simulink model "Tipo3_v4"  (R2018b)
settings: Solver=FixedStepDiscrete  StartTime=0.0  StopTime=30  MaxStep=50e-6  RelTol=1e-3
PreLoadFcn:
  | Ts=2e-6;
InitFcn:
  | %xInitial = init_power_wind_dfig_det;
  | Ts=2e-6;
undefined symbols (not defined in the file): D1, Delta, DiscIntNeverNeededParam, find_system, level
libraries: powerlib x142, simulink x110, powerlib_meascontrol x63, powerlib_extras x38, simulink_extras x10
(part 3 of 6)

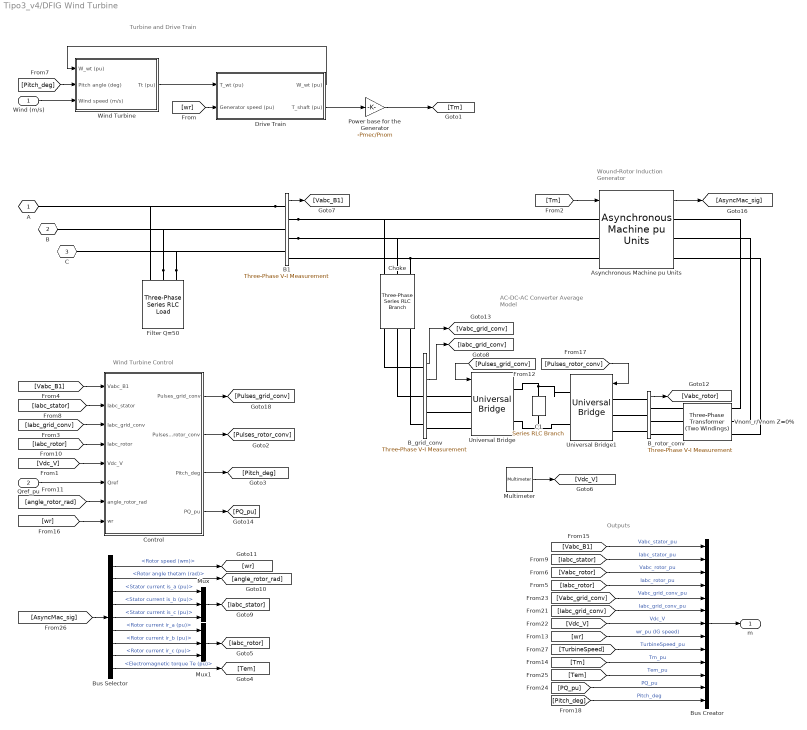
== system Tipo3_v4/DFIG Wind Turbine ==
  note: Turbine and Drive Train
  note: Wind Turbine Control
  note: Wound-Rotor
      | Induction Generator
  note: AC-DC-AC Converter
      | Average Model
  note: Outputs
  "Wind (m/s) " : Inport
  Qref_pu : Inport  Port=2
  Asynchronous Machine pu Units : powerlib/Machines/Asynchronous Machine pu Units  RotorType=Wound  PresetModel=No  MechanicalLoad=Torque Tm  ShowDetailedParameters=on  ReferenceFrame=Rotor  Units=pu  MeasurementBus=off  NominalParameters=[ Pnom Vnom Fnom ]  Stator=[ Rs Lls]  Rotor=[ Rr Llr]  Cage1=[0.01909 0.0397]  Cage2=[0.01909 0.0397]  Lm=Lm  Mechanical=[H F p]  PolePairs=3  InitialConditions=init  SimulateSaturation=off  Saturation="[0.212,0.4201,0.8125,1.0979,1.4799,2.2457,3.2586,4.5763,6.4763 ;   0.5,0.7,0.9,1,1.1,1.2 ,1.3,1.4,1.5]"  LoadFlowParameters=0  TsPowergui=0  TsBlock=-1  IterativeModel=Trapezoidal non iterative  IterativeDiscreteModel=Trapezoidal non iterative  Pmec=0
      settings: SourceProductName=Simscape Electrical  SourceProductBaseCode=PS
  B1 : powerlib/Measurements/Three-Phase V-I Measurement  VoltageMeasurement=phase-to-ground  SetLabelV=off  LabelV=Vabc  Vpu=on  VpuLL=off  CurrentMeasurement=no  SetLabelI=on  LabelI=Iabc_B1  Ipu=on  Pbase=Pnom  Vbase=Vnom  OutputType=Complex  PhasorSimulation=off  PSBequivalent=0
      settings: SourceProductName=Simscape Electrical
  B_grid_conv : powerlib/Measurements/Three-Phase V-I Measurement  VoltageMeasurement=phase-to-ground  SetLabelV=off  LabelV=Vabc_B1  Vpu=on  VpuLL=off  CurrentMeasurement=yes  SetLabelI=off  LabelI=Iabc  Ipu=on  Pbase=Pnom  Vbase=Vnom  OutputType=Complex  PhasorSimulation=off  PSBequivalent=0
      settings: SourceProductName=Simscape Electrical
  B_rotor_conv : powerlib/Measurements/Three-Phase V-I Measurement  VoltageMeasurement=phase-to-phase  SetLabelV=off  LabelV=Vabc_B1  Vpu=on  VpuLL=off  CurrentMeasurement=no  SetLabelI=off  LabelI=Iabc  Ipu=on  Pbase=Pnom  Vbase=Vnom_r  OutputType=Complex  PhasorSimulation=off  PSBequivalent=0
      settings: SourceProductName=Simscape Electrical
  Bus Creator : BusCreator  Inputs=13
  Bus Selector : BusSelector  OutputSignals=Mechanical.Rotor speed (wm),Mechanical.Rotor angle thetam (rad),Stator measurements.Stator current is_a (pu),Stator measurements.Stator current is_b (pu),Stator measurements.Stator current is_c (pu),Rotor measurements.Rotor current ir_a (pu),Rotor measurements.Rotor current ir_b (pu),Rotor measurements.Rotor current ir_c (pu),Mechanical.Electromagnetic torque Te (pu)
  C1 : powerlib/Elements/Series RLC Branch  LConnTagsString=__new0  RConnTagsString=__new0  BranchType=C  Resistance=[]  Inductance=[]  SetiL0=off  InitialCurrent=0  Capacitance=C_DClink  Setx0=on  InitialVoltage=Vdc_nom  Measurements=Branch voltage
      settings: SourceProductName=Simscape Electrical
  "Choke " : powerlib/Elements/Three-Phase Series RLC Branch  LConnTagsString=A|B|C  RConnTagsString=A|B|C  BranchType=RL  Resistance=R_RL*Vnom^2/Pnom  Inductance=L_RL*Vnom^2/Pnom/(2*pi*Fnom)  Capacitance=[]  Measurements=None
      settings: SourceProductName=Simscape Electrical
  Control : Subsystem
  Drive Train : Subsystem  mask(Wind Turbine shaft){H_WT=H_WT, Ksh=Ksh, D_mutual=D_mutual, wbase=2*pi*Fnom/p, w_wt0=w_wt0, torque0=torque0, Ts=Ts}
      mask prompts: H_WT "Wind turbine inertia constant H (s):"; Ksh "Shaft spring constant (pu of nominal mechanical torque/rad):"; D_mutual "Shaft mutual damping (pu of nominal mechanical torque/pu dw):"; wbase "Shaft base speed (rad/s):"; w_wt0 "Turbine initial speed (pu of base speed):"; torque0 "Initial output torque (pu of nominal mechanical torque):"; Ts "Sample time (s):"
      mask help:
      | This block implements a wind turbine drive train model. All shaft parameters are referred to high-speed shaft (generator shaft).
      |
      | The first input is the wind turbine torque in per unit (pu) based on the nominal power of the turbine and the base speed of the generator. The second input is the generator speed in pu based on the base speed of the generator.
      |
      | The outputs are:
      | 1- the transmitted torque of the shaft in pu based on the nominal power of the turbine and the base speed of the generator.
      | 2- the wind turbine speed in pu of the base speed of the generator.
  Filter Q=50 : powerlib/Elements/Three-Phase Series RLC Load  LConnTagsString=A|B|C  Configuration=Y (grounded)  NominalVoltage=Vnom  Vabc=[1e3 1e3 1e3]  Vabcp=[1e3 1e3 1e3]  NominalFrequency=Fnom  UnbalancedPower=off  ActivePower=C_var_filter/Q_filter  InductivePower=0  CapacitivePower=C_var_filter  Pabc=[10e3 9e3 11e3]  QLabc=[100 90 110]  QCabc=[100 90 110]  Pabcp=[10e3 9e3 11e3]  QLabcp=[100 90 110]  QCabcp=[100 90 110]  Measurements=None  LoadType=constant Z
      settings: SourceProductName=Simscape Electrical
  Multimeter : powerlib/Measurements/Multimeter  PhasorSimulation=off  OutputType=Complex  sel=1  L=1  Gain=1  yselected={'Ub: DFIG Wind Turbine/C1'};  PSBOutputType=1  PSBequivalent=0  AxesSetting=[0,0.1,-100,100]  Display=0  SavedBlockNames=-11
      settings: SourceProductName=Simscape Electrical
  Mux : Mux  Inputs=3
  Mux1 : Mux  Inputs=3
  Power base for the Generator : Gain  Gain=-Pmec/Pnom  SaturateOnIntegerOverflow=on  OutDataTypeStr=Inherit: Same as input  ParamDataTypeStr=Inherit: Same as input
  Universal Bridge : powerlib/Power Electronics/Universal Bridge  Arms=3  SnubberResistance=1e3  SnubberCapacitance=inf  Device=IGBT / Diodes  Ron=1e-4/Nb_wt  Lon=0  ForwardVoltages="[  0  0  ]"  ForwardVoltage=0  GTOparameters=[ 10e-6 , 20e-6 ]  IGBTparameters=[ 0 , 0 ]  Measurements=None  Measurements_2=None  converterType=Rectifier
      settings: SourceProductName=Simscape Electrical
  Universal Bridge1 : powerlib/Power Electronics/Universal Bridge  Arms=3  SnubberResistance=1e3  SnubberCapacitance=inf  Device=IGBT / Diodes  Ron=1e-4/Nb_wt  Lon=0  ForwardVoltages="[  0  0  ]"  ForwardVoltage=0  GTOparameters=[ 10e-6 , 20e-6 ]  IGBTparameters=[ 0 , 0 ]  Measurements=None  Measurements_2=None  converterType=Rectifier
      settings: SourceProductName=Simscape Electrical
  Vnom_r/Vnom Z=0% : powerlib/Elements/Three-Phase Transformer (Two Windings)  Winding1Connection=Y  Winding2Connection=Y  CoreType=Three single-phase transformers  SetSaturation=off  Hysteresis=off  DataFile='hysteresis'  SetInitialFlux=off  Measurements=None  UNITS=pu  NominalPower=[ Pnom , Fnom ]  Winding1=[ Vnom_r , 0, 0]  Winding2=[ Vnom , 0, 0]  Rm=500  Lm=inf  L0=0.5  Saturation=[ 0,0 ; 0.0024,1.2 ; 1.0,1.52 ]  InitialFluxes=[ 0.8 , -0.8 , 0.7 ]  MoreParameters=off  BreakLoop=off  DataType=off  TransfoNumber=0
      settings: SourceProductName=Simscape Electrical
  Wind Turbine : Subsystem  mask(Wind Turbine){Prated=Pmec, c1_c8=c1_c8, K1_K2=K1_K2, wind0=wind0, Ts=Ts}
      mask prompts: Prated "Nominal mechanical output power (W):"; c1_c8 "Coefficients [c1 ... c8]"; K1_K2 "Parameters [K1 K2]"; wind0 "Initial wind speed (m/s):"; Ts "Sample time (s):"
      mask help:
      | This block implements a generic wind turbine models.
      |
      | The first input is the turbine speed in per unit of the generator base speed. For a synchronous or asynchronous generator, the base speed is the synchronous speed. For a permanent-magnet generator, the base speed is defined as the speed producing nominal voltage at  no load. The second input is the blade pitch angle in degrees. The third input is the wind speed in m/s.
      |
      | The output is the torque applied to the drive train in per unit based on the nominal power of the turbine and the base speed of the generator.
      mask init:
      | c1 = c1_c8(1);
      | c2 = c1_c8(2);
      | c3 = c1_c8(3);
      | c4 = c1_c8(4);
      | c5 = c1_c8(5);
      | c6 = c1_c8(6);
      | c7 = c1_c8(7);;
      | c8 = c1_c8(8);
      | 
      | K1=K1_K2(1);
      | K2=K1_K2(2);
      settings: OpenFcn=power_openblockproxy();
      mask Display: disp('');
  A : PMIOPort  Tag=PMCPort  Side=Left
  B : PMIOPort  Tag=PMCPort  Port=2  Side=Left
  C : PMIOPort  Tag=PMCPort  Port=3  Side=Left
  m : Outport
  wires:
  [Pulses_rotor_conv] -> Universal Bridge1/1
  [Pulses_grid_conv] -> Universal Bridge/1
  Multimeter/1 -> [Vdc_V]
  [Pitch_deg] -> Bus Creator/13  "Pitch_deg"
  [PQ_pu] -> Bus Creator/12  "PQ_pu"
  Control/4(PQ_pu) -> [PQ_pu]
  [Tem] -> Bus Creator/11  "Tem_pu"
  [Tm] -> Bus Creator/10  "Tm_pu"
  [TurbineSpeed] -> Bus Creator/9  "TurbineSpeed_pu"
  [Vdc_V] -> Bus Creator/7  "Vdc_V"
  [Iabc_grid_conv] -> Bus Creator/6  "Iabc_grid_conv_pu"
  [Vabc_grid_conv] -> Bus Creator/5  "Vabc_grid_conv_pu"
  [Iabc_rotor] -> Bus Creator/4  "Iabc_rotor_pu"
  [Vabc_rotor] -> Bus Creator/3  "Vabc_rotor_pu"
  [Iabc_stator] -> Bus Creator/2  "Iabc_stator_pu"
  [Vabc_B1] -> Bus Creator/1  "Vabc_stator_pu"
  Asynchronous Machine pu Units/1 -> [AsyncMac_sig]
  Control/2(Pulses_rotor_conv) -> [Pulses_rotor_conv]
  [Pitch_deg] -> Wind Turbine/2(Pitch angle (deg))
  Drive Train/1(W_wt (pu)) -> Wind Turbine/1(W_wt (pu))
  "Wind (m/s) "/1 -> Wind Turbine/3(Wind speed (m/s))
  Power base for the Generator/1 -> [Tm]
  Drive Train/2(T_shaft (pu)) -> Power base for the Generator/1
  [wr] -> Drive Train/2(Generator speed (pu))
  Wind Turbine/1(Tt (pu)) -> Drive Train/1(T_wt (pu))
  Qref_pu/1 -> Control/6(Qref)
  Bus Selector/9 -> [Tem]  "<Electromagnetic torque Te (pu)>"
  Bus Selector/1 -> [wr]  "<Rotor speed (wm)>"
  Bus Creator/1 -> m/1
  B_rotor_conv/1 -> [Vabc_rotor]
  B1/1 -> [Vabc_B1]
  [Vabc_B1] -> Control/1(Vabc_B1)
  [Iabc_grid_conv] -> Control/3(Iabc_grid_conv)
  [Iabc_rotor] -> Control/4(Iabc_rotor)
  [angle_rotor_rad] -> Control/7(angle_rotor_rad)
  Mux1/1 -> [Iabc_rotor]
  Mux/1 -> [Iabc_stator]
  [Vdc_V] -> Control/5(Vdc_V)
  Control/3(Pitch_deg) -> [Pitch_deg]
  [Iabc_stator] -> Control/2(Iabc_stator)
  [wr] -> Control/8(wr)
  Bus Selector/8 -> Mux1/3  "<Rotor current ir_c (pu)>"
  Bus Selector/7 -> Mux1/2  "<Rotor current ir_b (pu)>"
  Bus Selector/6 -> Mux1/1  "<Rotor current ir_a (pu)>"
  Bus Selector/5 -> Mux/3  "<Stator current is_c (pu)>"
  Bus Selector/4 -> Mux/2  "<Stator current is_b (pu)>"
  Bus Selector/3 -> Mux/1  "<Stator current is_a (pu)>"
  Bus Selector/2 -> [angle_rotor_rad]  "<Rotor angle thetam (rad)>"
  B_grid_conv/2 -> [Iabc_grid_conv]
  B_grid_conv/1 -> [Vabc_grid_conv]
  Control/1(Pulses_grid_conv) -> [Pulses_grid_conv]
  [AsyncMac_sig] -> Bus Selector/1
  [wr] -> Bus Creator/8  "wr_pu (IG speed)"
  [Tm] -> Asynchronous Machine pu Units/1
  connections:
  Universal Bridge1/LConn3 -- B_rotor_conv/LConn3
  Universal Bridge1/LConn2 -- B_rotor_conv/LConn2
  Universal Bridge1/LConn1 -- B_rotor_conv/LConn1
  C1/LConn1 -- Universal Bridge/RConn1 -- Universal Bridge1/RConn1
  B_grid_conv/RConn2 -- Universal Bridge/LConn2
  B_grid_conv/RConn1 -- Universal Bridge/LConn1
  B_grid_conv/RConn3 -- Universal Bridge/LConn3
  C1/RConn1 -- Universal Bridge/RConn2 -- Universal Bridge1/RConn2
  Filter Q=50/LConn3 -- B1/LConn3 -- C/RConn1
  Filter Q=50/LConn2 -- B1/LConn2 -- B/RConn1
  B1/LConn1 -- Filter Q=50/LConn1 -- A/RConn1
  B_rotor_conv/RConn3 -- Vnom_r/Vnom Z=0%/LConn3
  B_rotor_conv/RConn2 -- Vnom_r/Vnom Z=0%/LConn2
  B_rotor_conv/RConn1 -- Vnom_r/Vnom Z=0%/LConn1
  B1/RConn3 -- "Choke "/LConn3 -- Asynchronous Machine pu Units/LConn3
  B1/RConn1 -- "Choke "/LConn1 -- Asynchronous Machine pu Units/LConn1
  Asynchronous Machine pu Units/RConn3 -- Vnom_r/Vnom Z=0%/RConn3
  Asynchronous Machine pu Units/RConn1 -- Vnom_r/Vnom Z=0%/RConn1
  Asynchronous Machine pu Units/RConn2 -- Vnom_r/Vnom Z=0%/RConn2
  "Choke "/RConn3 -- B_grid_conv/LConn3
  "Choke "/RConn2 -- B_grid_conv/LConn2
  "Choke "/RConn1 -- B_grid_conv/LConn1
  B1/RConn2 -- "Choke "/LConn2 -- Asynchronous Machine pu Units/LConn2

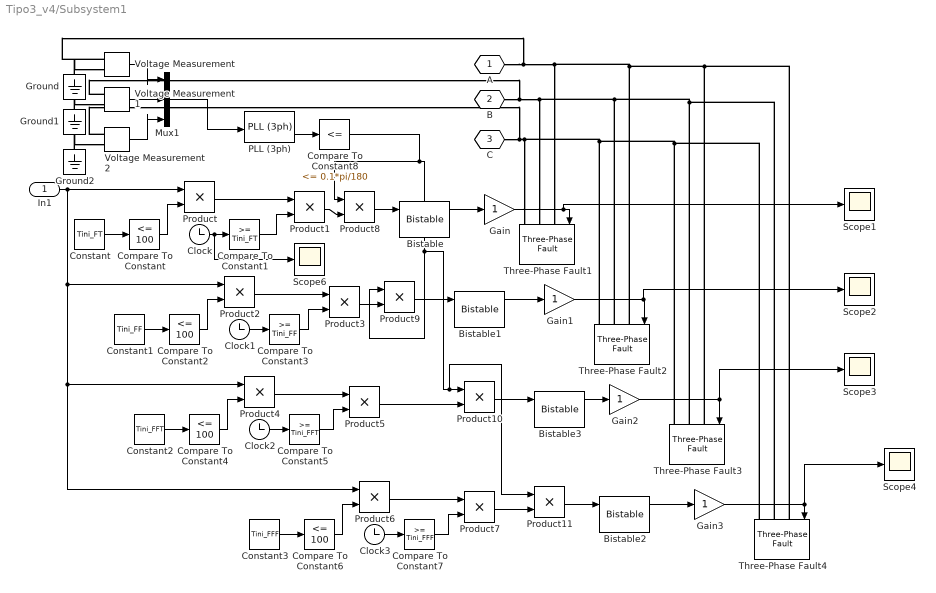
== system Tipo3_v4/Subsystem1 ==
  In1 : Inport
  Bistable{,1..3} (4 alike) : powerlib_meascontrol/Logic/Bistable  Qpriority=Set  ic=0  Ts=Ts
      settings: SourceProductName=Simscape Power Systems  SourceProductBaseCode=PS
  Clock{,1..3} (4 alike) : Clock
  Compare To Constant{,2,4,6} (4 alike) : simulink/Logic and Bit Operations/Compare To Constant  relop=<=  const=100  OutDataTypeStr=uint8
  Compare To Constant1 : simulink/Logic and Bit Operations/Compare To Constant  relop=>=  const=Tini_FT  OutDataTypeStr=uint8
  Compare To Constant3 : simulink/Logic and Bit Operations/Compare To Constant  relop=>=  const=Tini_FF  OutDataTypeStr=uint8
  Compare To Constant5 : simulink/Logic and Bit Operations/Compare To Constant  relop=>=  const=Tini_FFT  OutDataTypeStr=uint8
  Compare To Constant7 : simulink/Logic and Bit Operations/Compare To Constant  relop=>=  const=Tini_FFF  OutDataTypeStr=uint8
  Compare To Constant8 : simulink/Logic and Bit Operations/Compare To Constant  relop=<=  const=0.1*pi/180  OutDataTypeStr=uint8
  Constant : Constant  Value=Tini_FT
  Constant1 : Constant  Value=Tini_FF
  Constant2 : Constant  Value=Tini_FFT
  Constant3 : Constant  Value=Tini_FFF
  Gain{,1..3} (4 alike) : Gain  OutDataTypeStr=double
  Ground : powerlib/Elements/Ground  LConnTagsString=a
  Ground1 : powerlib/Elements/Ground  LConnTagsString=a
  Ground2 : powerlib/Elements/Ground  LConnTagsString=a
  Mux1 : Mux  Inputs=3
  PLL (3ph) : powerlib_meascontrol/PLL/PLL (3ph)  Fmin=60  Par_Init=[0, 60]  ParK=[180, 3200, 1]  TcD=1e-4  MaxRateChangeFreq=12  FilterCutOffFreq=25  Ts=Ts  AGC=on
  Product{,2..7} (7 alike) : Product
  Product{1,8..11} (5 alike) : Product  RndMeth=Ceiling
  Scope{1..4,6} (5 alike) : Scope
  Three-Phase Fault1 : powerlib/Elements/Three-Phase Fault  InitialStates=0  FaultA=on  FaultB=off  FaultC=off  GroundFault=on  SwitchTimes=[900 1000]  External=on  SwitchStatus=NaN  FaultResistance=R_falta  GroundResistance=R_falta  SnubberResistance=1e6  SnubberCapacitance=inf  Measurements=None
  Three-Phase Fault2 : powerlib/Elements/Three-Phase Fault  InitialStates=0  FaultA=on  FaultB=on  FaultC=off  GroundFault=off  SwitchTimes=[900 1000]  External=on  SwitchStatus=NaN  FaultResistance=R_falta  GroundResistance=1e-12  SnubberResistance=1e6  SnubberCapacitance=inf  Measurements=None
  Three-Phase Fault3 : powerlib/Elements/Three-Phase Fault  InitialStates=0  FaultA=on  FaultB=on  FaultC=off  GroundFault=on  SwitchTimes=[900 1000]  External=on  SwitchStatus=NaN  FaultResistance=R_falta  GroundResistance=R_falta  SnubberResistance=1e6  SnubberCapacitance=inf  Measurements=None
  Three-Phase Fault4 : powerlib/Elements/Three-Phase Fault  InitialStates=0  FaultA=on  FaultB=on  FaultC=on  GroundFault=on  SwitchTimes=[900 1000]  External=on  SwitchStatus=NaN  FaultResistance=R_falta  GroundResistance=R_falta  SnubberResistance=1e6  SnubberCapacitance=inf  Measurements=None
  Voltage Measurement : powerlib/Measurements/Voltage Measurement  PhasorSimulation=off  OutputType=Complex  PSBequivalent=0
  Voltage Measurement1 : powerlib/Measurements/Voltage Measurement  PhasorSimulation=off  OutputType=Complex  PSBequivalent=0
  Voltage Measurement2 : powerlib/Measurements/Voltage Measurement  PhasorSimulation=off  OutputType=Complex  PSBequivalent=0
  A : PMIOPort  Tag=PMCPort  Side=Right
  B : PMIOPort  Tag=PMCPort  Port=2  Side=Right
  C : PMIOPort  Tag=PMCPort  Port=3  Side=Right
  wires:
  Clock/1 -> Scope6/1, Compare To Constant1/1
  Product2/1 -> Product3/1
  Constant1/1 -> Compare To Constant2/1
  Product/1 -> Product1/1
  Compare To Constant2/1 -> Product2/2
  Constant2/1 -> Compare To Constant4/1
  Clock2/1 -> Compare To Constant5/1
  Compare To Constant4/1 -> Product4/2
  Clock1/1 -> Compare To Constant3/1
  Compare To Constant5/1 -> Product5/2
  In1/1 -> Product/1, Product2/1, Product4/1, Product6/1
  Clock3/1 -> Compare To Constant7/1
  Constant3/1 -> Compare To Constant6/1
  Compare To Constant6/1 -> Product6/2
  Product6/1 -> Product7/1
  Compare To Constant7/1 -> Product7/2
  Compare To Constant3/1 -> Product3/2
  Constant/1 -> Compare To Constant/1
  Compare To Constant/1 -> Product/2
  Compare To Constant1/1 -> Product1/2
  Product4/1 -> Product5/1
  Product1/1 -> Product8/2
  Product8/1 -> Bistable/1
  Product3/1 -> Product9/2
  Product5/1 -> Product10/2
  Product7/1 -> Product11/2
  Compare To Constant8/1 -> Product11/1, Product10/1, Product9/1, Product8/1
  PLL (3ph)/2 -> Compare To Constant8/1
  Voltage Measurement1/1 -> Mux1/2
  Voltage Measurement/1 -> Mux1/1
  Voltage Measurement2/1 -> Mux1/3
  Mux1/1 -> PLL (3ph)/1
  Gain/1 -> Scope1/1, Three-Phase Fault1/1
  Gain1/1 -> Scope2/1, Three-Phase Fault2/1
  Gain2/1 -> Three-Phase Fault3/1, Scope3/1
  Gain3/1 -> Scope4/1, Three-Phase Fault4/1
  Bistable/1 -> Gain/1
  Product9/1 -> Bistable1/1
  Bistable1/1 -> Gain1/1
  Bistable3/1 -> Gain2/1
  Product10/1 -> Bistable3/1
  Product11/1 -> Bistable2/1
  Bistable2/1 -> Gain3/1
  connections:
  Three-Phase Fault1/LConn2 -- Voltage Measurement1/LConn1 -- B/RConn1 -- Three-Phase Fault2/LConn2 -- Three-Phase Fault3/LConn2 -- Three-Phase Fault4/LConn2
  Three-Phase Fault1/LConn3 -- Voltage Measurement2/LConn1 -- C/RConn1 -- Three-Phase Fault4/LConn3 -- Three-Phase Fault3/LConn3 -- Three-Phase Fault2/LConn3
  A/RConn1 -- Voltage Measurement/LConn1 -- Three-Phase Fault2/LConn1 -- Three-Phase Fault3/LConn1 -- Three-Phase Fault4/LConn1 -- Three-Phase Fault1/LConn1
  Ground/LConn1 -- Voltage Measurement/LConn2
  Ground1/LConn1 -- Voltage Measurement1/LConn2
  Ground2/LConn1 -- Voltage Measurement2/LConn2

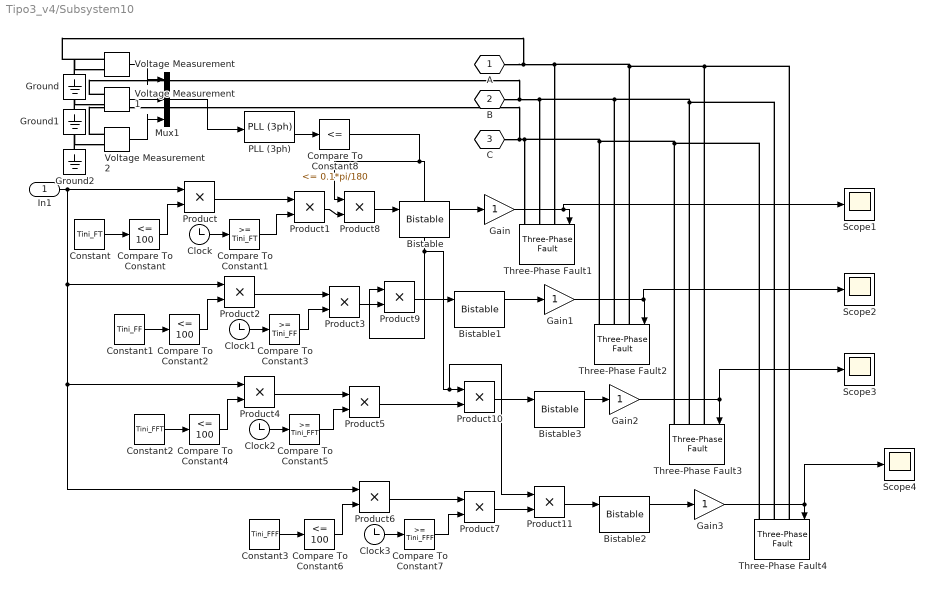
== system Tipo3_v4/Subsystem10 ==
  In1 : Inport
  Bistable{,1..3} (4 alike) : powerlib_meascontrol/Logic/Bistable  Qpriority=Set  ic=0  Ts=Ts
      settings: SourceProductName=Simscape Power Systems  SourceProductBaseCode=PS
  Clock{,1..3} (4 alike) : Clock
  Compare To Constant{,2,4,6} (4 alike) : simulink/Logic and Bit Operations/Compare To Constant  relop=<=  const=100  OutDataTypeStr=uint8
  Compare To Constant1 : simulink/Logic and Bit Operations/Compare To Constant  relop=>=  const=Tini_FT  OutDataTypeStr=uint8
  Compare To Constant3 : simulink/Logic and Bit Operations/Compare To Constant  relop=>=  const=Tini_FF  OutDataTypeStr=uint8
  Compare To Constant5 : simulink/Logic and Bit Operations/Compare To Constant  relop=>=  const=Tini_FFT  OutDataTypeStr=uint8
  Compare To Constant7 : simulink/Logic and Bit Operations/Compare To Constant  relop=>=  const=Tini_FFF  OutDataTypeStr=uint8
  Compare To Constant8 : simulink/Logic and Bit Operations/Compare To Constant  relop=<=  const=0.1*pi/180  OutDataTypeStr=uint8
  Constant : Constant  Value=Tini_FT
  Constant1 : Constant  Value=Tini_FF
  Constant2 : Constant  Value=Tini_FFT
  Constant3 : Constant  Value=Tini_FFF
  Gain{,1..3} (4 alike) : Gain  OutDataTypeStr=double
  Ground : powerlib/Elements/Ground  LConnTagsString=a
  Ground1 : powerlib/Elements/Ground  LConnTagsString=a
  Ground2 : powerlib/Elements/Ground  LConnTagsString=a
  Mux1 : Mux  Inputs=3
  PLL (3ph) : powerlib_meascontrol/PLL/PLL (3ph)  Fmin=60  Par_Init=[0, 60]  ParK=[180, 3200, 1]  TcD=1e-4  MaxRateChangeFreq=12  FilterCutOffFreq=25  Ts=Ts  AGC=on
  Product{,2..7} (7 alike) : Product
  Product{1,8..11} (5 alike) : Product  RndMeth=Ceiling
  Scope{1..4} (4 alike) : Scope
  Three-Phase Fault1 : powerlib/Elements/Three-Phase Fault  InitialStates=0  FaultA=on  FaultB=off  FaultC=off  GroundFault=on  SwitchTimes=[900 1000]  External=on  SwitchStatus=NaN  FaultResistance=R_falta  GroundResistance=R_falta  SnubberResistance=1e6  SnubberCapacitance=inf  Measurements=None
  Three-Phase Fault2 : powerlib/Elements/Three-Phase Fault  InitialStates=0  FaultA=on  FaultB=on  FaultC=off  GroundFault=off  SwitchTimes=[900 1000]  External=on  SwitchStatus=NaN  FaultResistance=R_falta  GroundResistance=1e-12  SnubberResistance=1e6  SnubberCapacitance=inf  Measurements=None
  Three-Phase Fault3 : powerlib/Elements/Three-Phase Fault  InitialStates=0  FaultA=on  FaultB=on  FaultC=off  GroundFault=on  SwitchTimes=[900 1000]  External=on  SwitchStatus=NaN  FaultResistance=R_falta  GroundResistance=R_falta  SnubberResistance=1e6  SnubberCapacitance=inf  Measurements=None
  Three-Phase Fault4 : powerlib/Elements/Three-Phase Fault  InitialStates=0  FaultA=on  FaultB=on  FaultC=on  GroundFault=on  SwitchTimes=[900 1000]  External=on  SwitchStatus=NaN  FaultResistance=R_falta  GroundResistance=R_falta  SnubberResistance=1e6  SnubberCapacitance=inf  Measurements=None
  Voltage Measurement : powerlib/Measurements/Voltage Measurement  PhasorSimulation=off  OutputType=Complex  PSBequivalent=0
  Voltage Measurement1 : powerlib/Measurements/Voltage Measurement  PhasorSimulation=off  OutputType=Complex  PSBequivalent=0
  Voltage Measurement2 : powerlib/Measurements/Voltage Measurement  PhasorSimulation=off  OutputType=Complex  PSBequivalent=0
  A : PMIOPort  Tag=PMCPort  Side=Right
  B : PMIOPort  Tag=PMCPort  Port=2  Side=Right
  C : PMIOPort  Tag=PMCPort  Port=3  Side=Right
  wires:
  Clock/1 -> Compare To Constant1/1
  Product2/1 -> Product3/1
  Constant1/1 -> Compare To Constant2/1
  Product/1 -> Product1/1
  Compare To Constant2/1 -> Product2/2
  Constant2/1 -> Compare To Constant4/1
  Clock2/1 -> Compare To Constant5/1
  Compare To Constant4/1 -> Product4/2
  Clock1/1 -> Compare To Constant3/1
  Compare To Constant5/1 -> Product5/2
  In1/1 -> Product/1, Product2/1, Product4/1, Product6/1
  Clock3/1 -> Compare To Constant7/1
  Constant3/1 -> Compare To Constant6/1
  Compare To Constant6/1 -> Product6/2
  Product6/1 -> Product7/1
  Compare To Constant7/1 -> Product7/2
  Compare To Constant3/1 -> Product3/2
  Constant/1 -> Compare To Constant/1
  Compare To Constant/1 -> Product/2
  Compare To Constant1/1 -> Product1/2
  Product4/1 -> Product5/1
  Product1/1 -> Product8/2
  Product8/1 -> Bistable/1
  Product3/1 -> Product9/2
  Product5/1 -> Product10/2
  Product7/1 -> Product11/2
  Compare To Constant8/1 -> Product11/1, Product10/1, Product9/1, Product8/1
  PLL (3ph)/2 -> Compare To Constant8/1
  Voltage Measurement1/1 -> Mux1/2
  Voltage Measurement/1 -> Mux1/1
  Voltage Measurement2/1 -> Mux1/3
  Mux1/1 -> PLL (3ph)/1
  Gain/1 -> Scope1/1, Three-Phase Fault1/1
  Gain1/1 -> Scope2/1, Three-Phase Fault2/1
  Gain2/1 -> Three-Phase Fault3/1, Scope3/1
  Gain3/1 -> Scope4/1, Three-Phase Fault4/1
  Bistable/1 -> Gain/1
  Product9/1 -> Bistable1/1
  Bistable1/1 -> Gain1/1
  Bistable3/1 -> Gain2/1
  Product10/1 -> Bistable3/1
  Product11/1 -> Bistable2/1
  Bistable2/1 -> Gain3/1
  connections:
  Voltage Measurement1/LConn1 -- B/RConn1 -- Three-Phase Fault1/LConn2 -- Three-Phase Fault2/LConn2 -- Three-Phase Fault3/LConn2 -- Three-Phase Fault4/LConn2
  Voltage Measurement2/LConn1 -- C/RConn1 -- Three-Phase Fault4/LConn3 -- Three-Phase Fault3/LConn3 -- Three-Phase Fault2/LConn3 -- Three-Phase Fault1/LConn3
  A/RConn1 -- Voltage Measurement/LConn1 -- Three-Phase Fault1/LConn1 -- Three-Phase Fault2/LConn1 -- Three-Phase Fault3/LConn1 -- Three-Phase Fault4/LConn1
  Ground/LConn1 -- Voltage Measurement/LConn2
  Ground1/LConn1 -- Voltage Measurement1/LConn2
  Ground2/LConn1 -- Voltage Measurement2/LConn2

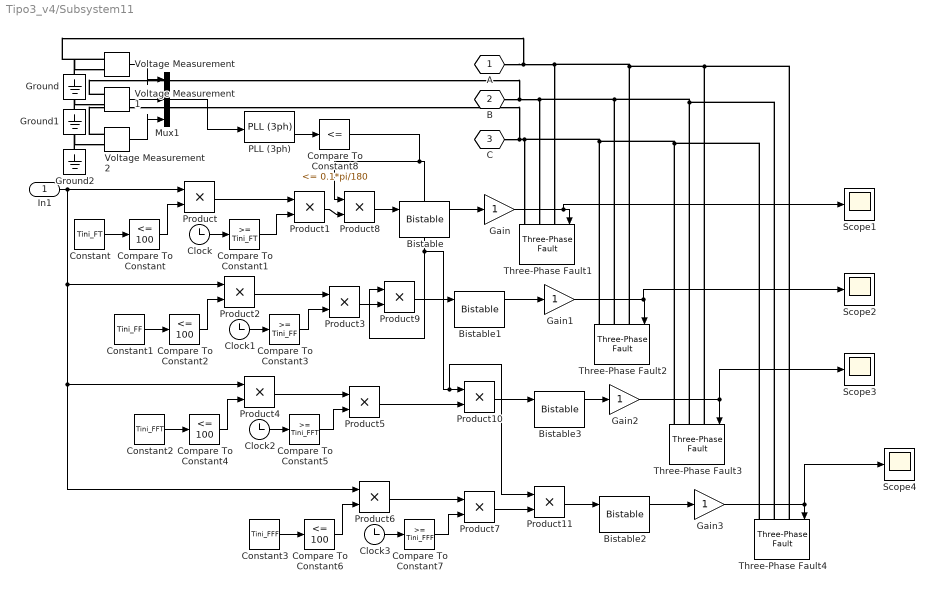
== system Tipo3_v4/Subsystem11 ==
  In1 : Inport
  Bistable{,1..3} (4 alike) : powerlib_meascontrol/Logic/Bistable  Qpriority=Set  ic=0  Ts=Ts
      settings: SourceProductName=Simscape Power Systems  SourceProductBaseCode=PS
  Clock{,1..3} (4 alike) : Clock
  Compare To Constant{,2,4,6} (4 alike) : simulink/Logic and Bit Operations/Compare To Constant  relop=<=  const=100  OutDataTypeStr=uint8
  Compare To Constant1 : simulink/Logic and Bit Operations/Compare To Constant  relop=>=  const=Tini_FT  OutDataTypeStr=uint8
  Compare To Constant3 : simulink/Logic and Bit Operations/Compare To Constant  relop=>=  const=Tini_FF  OutDataTypeStr=uint8
  Compare To Constant5 : simulink/Logic and Bit Operations/Compare To Constant  relop=>=  const=Tini_FFT  OutDataTypeStr=uint8
  Compare To Constant7 : simulink/Logic and Bit Operations/Compare To Constant  relop=>=  const=Tini_FFF  OutDataTypeStr=uint8
  Compare To Constant8 : simulink/Logic and Bit Operations/Compare To Constant  relop=<=  const=0.1*pi/180  OutDataTypeStr=uint8
  Constant : Constant  Value=Tini_FT
  Constant1 : Constant  Value=Tini_FF
  Constant2 : Constant  Value=Tini_FFT
  Constant3 : Constant  Value=Tini_FFF
  Gain{,1..3} (4 alike) : Gain  OutDataTypeStr=double
  Ground : powerlib/Elements/Ground  LConnTagsString=a
  Ground1 : powerlib/Elements/Ground  LConnTagsString=a
  Ground2 : powerlib/Elements/Ground  LConnTagsString=a
  Mux1 : Mux  Inputs=3
  PLL (3ph) : powerlib_meascontrol/PLL/PLL (3ph)  Fmin=60  Par_Init=[0, 60]  ParK=[180, 3200, 1]  TcD=1e-4  MaxRateChangeFreq=12  FilterCutOffFreq=25  Ts=Ts  AGC=on
  Product{,2..7} (7 alike) : Product
  Product{1,8..11} (5 alike) : Product  RndMeth=Ceiling
  Scope{1..4} (4 alike) : Scope
  Three-Phase Fault1 : powerlib/Elements/Three-Phase Fault  InitialStates=0  FaultA=on  FaultB=off  FaultC=off  GroundFault=on  SwitchTimes=[900 1000]  External=on  SwitchStatus=NaN  FaultResistance=R_falta  GroundResistance=R_falta  SnubberResistance=1e6  SnubberCapacitance=inf  Measurements=None
  Three-Phase Fault2 : powerlib/Elements/Three-Phase Fault  InitialStates=0  FaultA=on  FaultB=on  FaultC=off  GroundFault=off  SwitchTimes=[900 1000]  External=on  SwitchStatus=NaN  FaultResistance=R_falta  GroundResistance=1e-12  SnubberResistance=1e6  SnubberCapacitance=inf  Measurements=None
  Three-Phase Fault3 : powerlib/Elements/Three-Phase Fault  InitialStates=0  FaultA=on  FaultB=on  FaultC=off  GroundFault=on  SwitchTimes=[900 1000]  External=on  SwitchStatus=NaN  FaultResistance=R_falta  GroundResistance=R_falta  SnubberResistance=1e6  SnubberCapacitance=inf  Measurements=None
  Three-Phase Fault4 : powerlib/Elements/Three-Phase Fault  InitialStates=0  FaultA=on  FaultB=on  FaultC=on  GroundFault=on  SwitchTimes=[900 1000]  External=on  SwitchStatus=NaN  FaultResistance=R_falta  GroundResistance=R_falta  SnubberResistance=1e6  SnubberCapacitance=inf  Measurements=None
  Voltage Measurement : powerlib/Measurements/Voltage Measurement  PhasorSimulation=off  OutputType=Complex  PSBequivalent=0
  Voltage Measurement1 : powerlib/Measurements/Voltage Measurement  PhasorSimulation=off  OutputType=Complex  PSBequivalent=0
  Voltage Measurement2 : powerlib/Measurements/Voltage Measurement  PhasorSimulation=off  OutputType=Complex  PSBequivalent=0
  A : PMIOPort  Tag=PMCPort  Side=Right
  B : PMIOPort  Tag=PMCPort  Port=2  Side=Right
  C : PMIOPort  Tag=PMCPort  Port=3  Side=Right
  wires:
  Clock/1 -> Compare To Constant1/1
  Product2/1 -> Product3/1
  Constant1/1 -> Compare To Constant2/1
  Product/1 -> Product1/1
  Compare To Constant2/1 -> Product2/2
  Constant2/1 -> Compare To Constant4/1
  Clock2/1 -> Compare To Constant5/1
  Compare To Constant4/1 -> Product4/2
  Clock1/1 -> Compare To Constant3/1
  Compare To Constant5/1 -> Product5/2
  In1/1 -> Product/1, Product2/1, Product4/1, Product6/1
  Clock3/1 -> Compare To Constant7/1
  Constant3/1 -> Compare To Constant6/1
  Compare To Constant6/1 -> Product6/2
  Product6/1 -> Product7/1
  Compare To Constant7/1 -> Product7/2
  Compare To Constant3/1 -> Product3/2
  Constant/1 -> Compare To Constant/1
  Compare To Constant/1 -> Product/2
  Compare To Constant1/1 -> Product1/2
  Product4/1 -> Product5/1
  Product1/1 -> Product8/2
  Product8/1 -> Bistable/1
  Product3/1 -> Product9/2
  Product5/1 -> Product10/2
  Product7/1 -> Product11/2
  Compare To Constant8/1 -> Product11/1, Product10/1, Product9/1, Product8/1
  PLL (3ph)/2 -> Compare To Constant8/1
  Voltage Measurement1/1 -> Mux1/2
  Voltage Measurement/1 -> Mux1/1
  Voltage Measurement2/1 -> Mux1/3
  Mux1/1 -> PLL (3ph)/1
  Gain/1 -> Scope1/1, Three-Phase Fault1/1
  Gain1/1 -> Scope2/1, Three-Phase Fault2/1
  Gain2/1 -> Three-Phase Fault3/1, Scope3/1
  Gain3/1 -> Scope4/1, Three-Phase Fault4/1
  Bistable/1 -> Gain/1
  Product9/1 -> Bistable1/1
  Bistable1/1 -> Gain1/1
  Bistable3/1 -> Gain2/1
  Product10/1 -> Bistable3/1
  Product11/1 -> Bistable2/1
  Bistable2/1 -> Gain3/1
  connections:
  Voltage Measurement1/LConn1 -- B/RConn1 -- Three-Phase Fault1/LConn2 -- Three-Phase Fault2/LConn2 -- Three-Phase Fault3/LConn2 -- Three-Phase Fault4/LConn2
  Voltage Measurement2/LConn1 -- C/RConn1 -- Three-Phase Fault4/LConn3 -- Three-Phase Fault3/LConn3 -- Three-Phase Fault2/LConn3 -- Three-Phase Fault1/LConn3
  A/RConn1 -- Voltage Measurement/LConn1 -- Three-Phase Fault1/LConn1 -- Three-Phase Fault2/LConn1 -- Three-Phase Fault3/LConn1 -- Three-Phase Fault4/LConn1
  Ground/LConn1 -- Voltage Measurement/LConn2
  Ground1/LConn1 -- Voltage Measurement1/LConn2
  Ground2/LConn1 -- Voltage Measurement2/LConn2

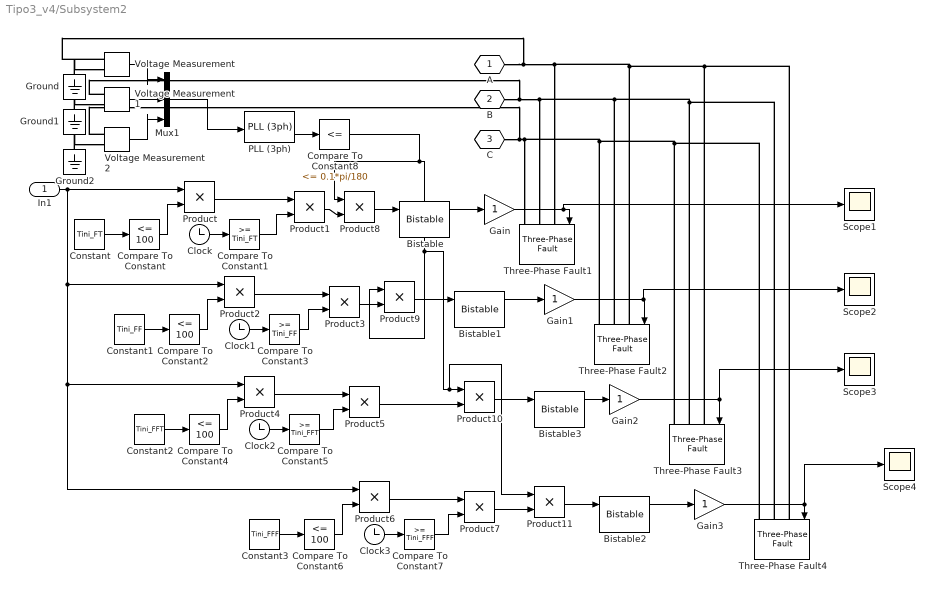
== system Tipo3_v4/Subsystem2 ==
  In1 : Inport
  Bistable{,1..3} (4 alike) : powerlib_meascontrol/Logic/Bistable  Qpriority=Set  ic=0  Ts=Ts
      settings: SourceProductName=Simscape Power Systems  SourceProductBaseCode=PS
  Clock{,1..3} (4 alike) : Clock
  Compare To Constant{,2,4,6} (4 alike) : simulink/Logic and Bit Operations/Compare To Constant  relop=<=  const=100  OutDataTypeStr=uint8
  Compare To Constant1 : simulink/Logic and Bit Operations/Compare To Constant  relop=>=  const=Tini_FT  OutDataTypeStr=uint8
  Compare To Constant3 : simulink/Logic and Bit Operations/Compare To Constant  relop=>=  const=Tini_FF  OutDataTypeStr=uint8
  Compare To Constant5 : simulink/Logic and Bit Operations/Compare To Constant  relop=>=  const=Tini_FFT  OutDataTypeStr=uint8
  Compare To Constant7 : simulink/Logic and Bit Operations/Compare To Constant  relop=>=  const=Tini_FFF  OutDataTypeStr=uint8
  Compare To Constant8 : simulink/Logic and Bit Operations/Compare To Constant  relop=<=  const=0.1*pi/180  OutDataTypeStr=uint8
  Constant : Constant  Value=Tini_FT
  Constant1 : Constant  Value=Tini_FF
  Constant2 : Constant  Value=Tini_FFT
  Constant3 : Constant  Value=Tini_FFF
  Gain{,1..3} (4 alike) : Gain  OutDataTypeStr=double
  Ground : powerlib/Elements/Ground  LConnTagsString=a
  Ground1 : powerlib/Elements/Ground  LConnTagsString=a
  Ground2 : powerlib/Elements/Ground  LConnTagsString=a
  Mux1 : Mux  Inputs=3
  PLL (3ph) : powerlib_meascontrol/PLL/PLL (3ph)  Fmin=60  Par_Init=[0, 60]  ParK=[180, 3200, 1]  TcD=1e-4  MaxRateChangeFreq=12  FilterCutOffFreq=25  Ts=Ts  AGC=on
  Product{,2..7} (7 alike) : Product
  Product{1,8..11} (5 alike) : Product  RndMeth=Ceiling
  Scope{1..4} (4 alike) : Scope
  Three-Phase Fault1 : powerlib/Elements/Three-Phase Fault  InitialStates=0  FaultA=on  FaultB=off  FaultC=off  GroundFault=on  SwitchTimes=[900 1000]  External=on  SwitchStatus=NaN  FaultResistance=R_falta  GroundResistance=R_falta  SnubberResistance=1e6  SnubberCapacitance=inf  Measurements=None
  Three-Phase Fault2 : powerlib/Elements/Three-Phase Fault  InitialStates=0  FaultA=on  FaultB=on  FaultC=off  GroundFault=off  SwitchTimes=[900 1000]  External=on  SwitchStatus=NaN  FaultResistance=R_falta  GroundResistance=1e-12  SnubberResistance=1e6  SnubberCapacitance=inf  Measurements=None
  Three-Phase Fault3 : powerlib/Elements/Three-Phase Fault  InitialStates=0  FaultA=on  FaultB=on  FaultC=off  GroundFault=on  SwitchTimes=[900 1000]  External=on  SwitchStatus=NaN  FaultResistance=R_falta  GroundResistance=R_falta  SnubberResistance=1e6  SnubberCapacitance=inf  Measurements=None
  Three-Phase Fault4 : powerlib/Elements/Three-Phase Fault  InitialStates=0  FaultA=on  FaultB=on  FaultC=on  GroundFault=on  SwitchTimes=[900 1000]  External=on  SwitchStatus=NaN  FaultResistance=R_falta  GroundResistance=R_falta  SnubberResistance=1e6  SnubberCapacitance=inf  Measurements=None
  Voltage Measurement : powerlib/Measurements/Voltage Measurement  PhasorSimulation=off  OutputType=Complex  PSBequivalent=0
  Voltage Measurement1 : powerlib/Measurements/Voltage Measurement  PhasorSimulation=off  OutputType=Complex  PSBequivalent=0
  Voltage Measurement2 : powerlib/Measurements/Voltage Measurement  PhasorSimulation=off  OutputType=Complex  PSBequivalent=0
  A : PMIOPort  Tag=PMCPort  Side=Right
  B : PMIOPort  Tag=PMCPort  Port=2  Side=Right
  C : PMIOPort  Tag=PMCPort  Port=3  Side=Right
  wires:
  Clock/1 -> Compare To Constant1/1
  Product2/1 -> Product3/1
  Constant1/1 -> Compare To Constant2/1
  Product/1 -> Product1/1
  Compare To Constant2/1 -> Product2/2
  Constant2/1 -> Compare To Constant4/1
  Clock2/1 -> Compare To Constant5/1
  Compare To Constant4/1 -> Product4/2
  Clock1/1 -> Compare To Constant3/1
  Compare To Constant5/1 -> Product5/2
  In1/1 -> Product/1, Product2/1, Product4/1, Product6/1
  Clock3/1 -> Compare To Constant7/1
  Constant3/1 -> Compare To Constant6/1
  Compare To Constant6/1 -> Product6/2
  Product6/1 -> Product7/1
  Compare To Constant7/1 -> Product7/2
  Compare To Constant3/1 -> Product3/2
  Constant/1 -> Compare To Constant/1
  Compare To Constant/1 -> Product/2
  Compare To Constant1/1 -> Product1/2
  Product4/1 -> Product5/1
  Product1/1 -> Product8/2
  Product8/1 -> Bistable/1
  Product3/1 -> Product9/2
  Product5/1 -> Product10/2
  Product7/1 -> Product11/2
  Compare To Constant8/1 -> Product11/1, Product10/1, Product9/1, Product8/1
  PLL (3ph)/2 -> Compare To Constant8/1
  Voltage Measurement1/1 -> Mux1/2
  Voltage Measurement/1 -> Mux1/1
  Voltage Measurement2/1 -> Mux1/3
  Mux1/1 -> PLL (3ph)/1
  Gain/1 -> Scope1/1, Three-Phase Fault1/1
  Gain1/1 -> Scope2/1, Three-Phase Fault2/1
  Gain2/1 -> Three-Phase Fault3/1, Scope3/1
  Gain3/1 -> Scope4/1, Three-Phase Fault4/1
  Bistable/1 -> Gain/1
  Product9/1 -> Bistable1/1
  Bistable1/1 -> Gain1/1
  Bistable3/1 -> Gain2/1
  Product10/1 -> Bistable3/1
  Product11/1 -> Bistable2/1
  Bistable2/1 -> Gain3/1
  connections:
  Voltage Measurement1/LConn1 -- B/RConn1 -- Three-Phase Fault1/LConn2 -- Three-Phase Fault2/LConn2 -- Three-Phase Fault3/LConn2 -- Three-Phase Fault4/LConn2
  Voltage Measurement2/LConn1 -- C/RConn1 -- Three-Phase Fault4/LConn3 -- Three-Phase Fault3/LConn3 -- Three-Phase Fault2/LConn3 -- Three-Phase Fault1/LConn3
  A/RConn1 -- Voltage Measurement/LConn1 -- Three-Phase Fault1/LConn1 -- Three-Phase Fault2/LConn1 -- Three-Phase Fault3/LConn1 -- Three-Phase Fault4/LConn1
  Ground/LConn1 -- Voltage Measurement/LConn2
  Ground1/LConn1 -- Voltage Measurement1/LConn2
  Ground2/LConn1 -- Voltage Measurement2/LConn2

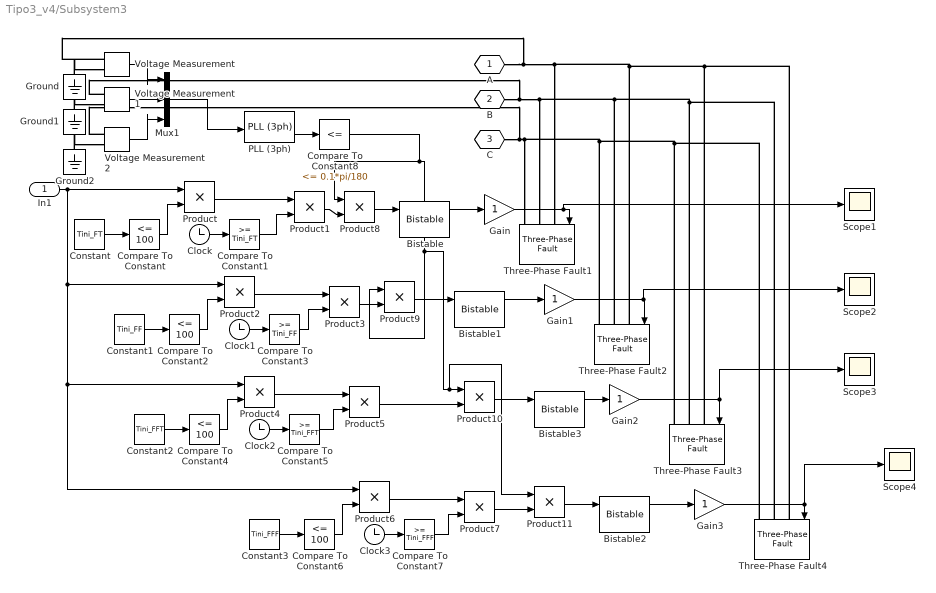
== system Tipo3_v4/Subsystem3 ==
  In1 : Inport
  Bistable{,1..3} (4 alike) : powerlib_meascontrol/Logic/Bistable  Qpriority=Set  ic=0  Ts=Ts
      settings: SourceProductName=Simscape Power Systems  SourceProductBaseCode=PS
  Clock{,1..3} (4 alike) : Clock
  Compare To Constant{,2,4,6} (4 alike) : simulink/Logic and Bit Operations/Compare To Constant  relop=<=  const=100  OutDataTypeStr=uint8
  Compare To Constant1 : simulink/Logic and Bit Operations/Compare To Constant  relop=>=  const=Tini_FT  OutDataTypeStr=uint8
  Compare To Constant3 : simulink/Logic and Bit Operations/Compare To Constant  relop=>=  const=Tini_FF  OutDataTypeStr=uint8
  Compare To Constant5 : simulink/Logic and Bit Operations/Compare To Constant  relop=>=  const=Tini_FFT  OutDataTypeStr=uint8
  Compare To Constant7 : simulink/Logic and Bit Operations/Compare To Constant  relop=>=  const=Tini_FFF  OutDataTypeStr=uint8
  Compare To Constant8 : simulink/Logic and Bit Operations/Compare To Constant  relop=<=  const=0.1*pi/180  OutDataTypeStr=uint8
  Constant : Constant  Value=Tini_FT
  Constant1 : Constant  Value=Tini_FF
  Constant2 : Constant  Value=Tini_FFT
  Constant3 : Constant  Value=Tini_FFF
  Gain{,1..3} (4 alike) : Gain  OutDataTypeStr=double
  Ground : powerlib/Elements/Ground  LConnTagsString=a
  Ground1 : powerlib/Elements/Ground  LConnTagsString=a
  Ground2 : powerlib/Elements/Ground  LConnTagsString=a
  Mux1 : Mux  Inputs=3
  PLL (3ph) : powerlib_meascontrol/PLL/PLL (3ph)  Fmin=60  Par_Init=[0, 60]  ParK=[180, 3200, 1]  TcD=1e-4  MaxRateChangeFreq=12  FilterCutOffFreq=25  Ts=Ts  AGC=on
  Product{,2..7} (7 alike) : Product
  Product{1,8..11} (5 alike) : Product  RndMeth=Ceiling
  Scope{1..4} (4 alike) : Scope
  Three-Phase Fault1 : powerlib/Elements/Three-Phase Fault  InitialStates=0  FaultA=on  FaultB=off  FaultC=off  GroundFault=on  SwitchTimes=[900 1000]  External=on  SwitchStatus=NaN  FaultResistance=R_falta  GroundResistance=R_falta  SnubberResistance=1e6  SnubberCapacitance=inf  Measurements=None
  Three-Phase Fault2 : powerlib/Elements/Three-Phase Fault  InitialStates=0  FaultA=on  FaultB=on  FaultC=off  GroundFault=off  SwitchTimes=[900 1000]  External=on  SwitchStatus=NaN  FaultResistance=R_falta  GroundResistance=1e-12  SnubberResistance=1e6  SnubberCapacitance=inf  Measurements=None
  Three-Phase Fault3 : powerlib/Elements/Three-Phase Fault  InitialStates=0  FaultA=on  FaultB=on  FaultC=off  GroundFault=on  SwitchTimes=[900 1000]  External=on  SwitchStatus=NaN  FaultResistance=R_falta  GroundResistance=R_falta  SnubberResistance=1e6  SnubberCapacitance=inf  Measurements=None
  Three-Phase Fault4 : powerlib/Elements/Three-Phase Fault  InitialStates=0  FaultA=on  FaultB=on  FaultC=on  GroundFault=on  SwitchTimes=[900 1000]  External=on  SwitchStatus=NaN  FaultResistance=R_falta  GroundResistance=R_falta  SnubberResistance=1e6  SnubberCapacitance=inf  Measurements=None
  Voltage Measurement : powerlib/Measurements/Voltage Measurement  PhasorSimulation=off  OutputType=Complex  PSBequivalent=0
  Voltage Measurement1 : powerlib/Measurements/Voltage Measurement  PhasorSimulation=off  OutputType=Complex  PSBequivalent=0
  Voltage Measurement2 : powerlib/Measurements/Voltage Measurement  PhasorSimulation=off  OutputType=Complex  PSBequivalent=0
  A : PMIOPort  Tag=PMCPort  Side=Right
  B : PMIOPort  Tag=PMCPort  Port=2  Side=Right
  C : PMIOPort  Tag=PMCPort  Port=3  Side=Right
  wires:
  Clock/1 -> Compare To Constant1/1
  Product2/1 -> Product3/1
  Constant1/1 -> Compare To Constant2/1
  Product/1 -> Product1/1
  Compare To Constant2/1 -> Product2/2
  Constant2/1 -> Compare To Constant4/1
  Clock2/1 -> Compare To Constant5/1
  Compare To Constant4/1 -> Product4/2
  Clock1/1 -> Compare To Constant3/1
  Compare To Constant5/1 -> Product5/2
  In1/1 -> Product/1, Product2/1, Product4/1, Product6/1
  Clock3/1 -> Compare To Constant7/1
  Constant3/1 -> Compare To Constant6/1
  Compare To Constant6/1 -> Product6/2
  Product6/1 -> Product7/1
  Compare To Constant7/1 -> Product7/2
  Compare To Constant3/1 -> Product3/2
  Constant/1 -> Compare To Constant/1
  Compare To Constant/1 -> Product/2
  Compare To Constant1/1 -> Product1/2
  Product4/1 -> Product5/1
  Product1/1 -> Product8/2
  Product8/1 -> Bistable/1
  Product3/1 -> Product9/2
  Product5/1 -> Product10/2
  Product7/1 -> Product11/2
  Compare To Constant8/1 -> Product11/1, Product10/1, Product9/1, Product8/1
  PLL (3ph)/2 -> Compare To Constant8/1
  Voltage Measurement1/1 -> Mux1/2
  Voltage Measurement/1 -> Mux1/1
  Voltage Measurement2/1 -> Mux1/3
  Mux1/1 -> PLL (3ph)/1
  Gain/1 -> Scope1/1, Three-Phase Fault1/1
  Gain1/1 -> Scope2/1, Three-Phase Fault2/1
  Gain2/1 -> Three-Phase Fault3/1, Scope3/1
  Gain3/1 -> Scope4/1, Three-Phase Fault4/1
  Bistable/1 -> Gain/1
  Product9/1 -> Bistable1/1
  Bistable1/1 -> Gain1/1
  Bistable3/1 -> Gain2/1
  Product10/1 -> Bistable3/1
  Product11/1 -> Bistable2/1
  Bistable2/1 -> Gain3/1
  connections:
  Voltage Measurement1/LConn1 -- B/RConn1 -- Three-Phase Fault1/LConn2 -- Three-Phase Fault2/LConn2 -- Three-Phase Fault3/LConn2 -- Three-Phase Fault4/LConn2
  Voltage Measurement2/LConn1 -- C/RConn1 -- Three-Phase Fault4/LConn3 -- Three-Phase Fault3/LConn3 -- Three-Phase Fault2/LConn3 -- Three-Phase Fault1/LConn3
  A/RConn1 -- Voltage Measurement/LConn1 -- Three-Phase Fault1/LConn1 -- Three-Phase Fault2/LConn1 -- Three-Phase Fault3/LConn1 -- Three-Phase Fault4/LConn1
  Ground/LConn1 -- Voltage Measurement/LConn2
  Ground1/LConn1 -- Voltage Measurement1/LConn2
  Ground2/LConn1 -- Voltage Measurement2/LConn2

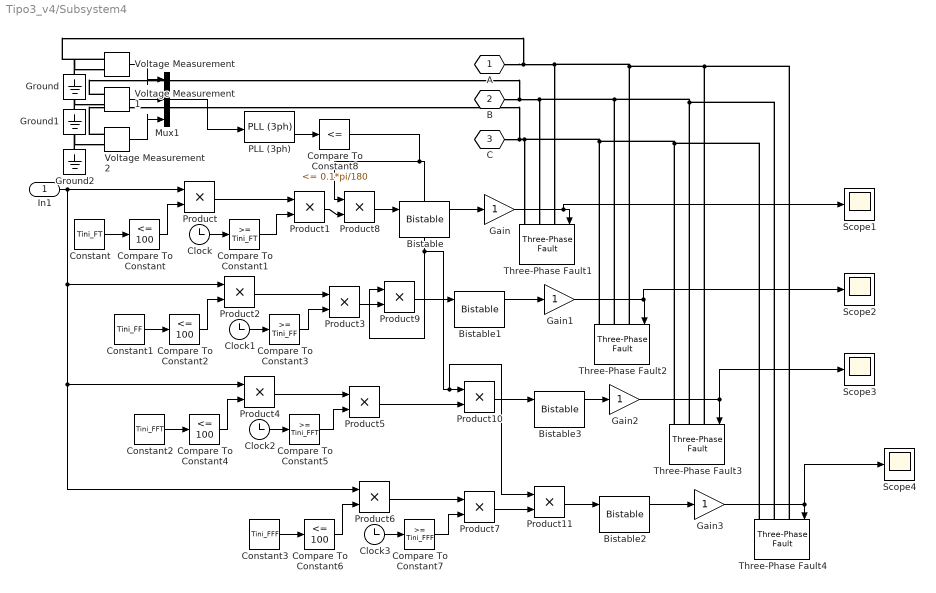
== system Tipo3_v4/Subsystem4 ==
  In1 : Inport
  Bistable{,1..3} (4 alike) : powerlib_meascontrol/Logic/Bistable  Qpriority=Set  ic=0  Ts=Ts
      settings: SourceProductName=Simscape Power Systems  SourceProductBaseCode=PS
  Clock{,1..3} (4 alike) : Clock
  Compare To Constant{,2,4,6} (4 alike) : simulink/Logic and Bit Operations/Compare To Constant  relop=<=  const=100  OutDataTypeStr=uint8
  Compare To Constant1 : simulink/Logic and Bit Operations/Compare To Constant  relop=>=  const=Tini_FT  OutDataTypeStr=uint8
  Compare To Constant3 : simulink/Logic and Bit Operations/Compare To Constant  relop=>=  const=Tini_FF  OutDataTypeStr=uint8
  Compare To Constant5 : simulink/Logic and Bit Operations/Compare To Constant  relop=>=  const=Tini_FFT  OutDataTypeStr=uint8
  Compare To Constant7 : simulink/Logic and Bit Operations/Compare To Constant  relop=>=  const=Tini_FFF  OutDataTypeStr=uint8
  Compare To Constant8 : simulink/Logic and Bit Operations/Compare To Constant  relop=<=  const=0.1*pi/180  OutDataTypeStr=uint8
  Constant : Constant  Value=Tini_FT
  Constant1 : Constant  Value=Tini_FF
  Constant2 : Constant  Value=Tini_FFT
  Constant3 : Constant  Value=Tini_FFF
  Gain{,1..3} (4 alike) : Gain  OutDataTypeStr=double
  Ground : powerlib/Elements/Ground  LConnTagsString=a
  Ground1 : powerlib/Elements/Ground  LConnTagsString=a
  Ground2 : powerlib/Elements/Ground  LConnTagsString=a
  Mux1 : Mux  Inputs=3
  PLL (3ph) : powerlib_meascontrol/PLL/PLL (3ph)  Fmin=60  Par_Init=[0, 60]  ParK=[180, 3200, 1]  TcD=1e-4  MaxRateChangeFreq=12  FilterCutOffFreq=25  Ts=Ts  AGC=on
  Product{,2..7} (7 alike) : Product
  Product{1,8..11} (5 alike) : Product  RndMeth=Ceiling
  Scope{1..4} (4 alike) : Scope
  Three-Phase Fault1 : powerlib/Elements/Three-Phase Fault  InitialStates=0  FaultA=on  FaultB=off  FaultC=off  GroundFault=on  SwitchTimes=[900 1000]  External=on  SwitchStatus=NaN  FaultResistance=R_falta  GroundResistance=R_falta  SnubberResistance=1e6  SnubberCapacitance=inf  Measurements=None
  Three-Phase Fault2 : powerlib/Elements/Three-Phase Fault  InitialStates=0  FaultA=on  FaultB=on  FaultC=off  GroundFault=off  SwitchTimes=[900 1000]  External=on  SwitchStatus=NaN  FaultResistance=R_falta  GroundResistance=1e-12  SnubberResistance=1e6  SnubberCapacitance=inf  Measurements=None
  Three-Phase Fault3 : powerlib/Elements/Three-Phase Fault  InitialStates=0  FaultA=on  FaultB=on  FaultC=off  GroundFault=on  SwitchTimes=[900 1000]  External=on  SwitchStatus=NaN  FaultResistance=R_falta  GroundResistance=R_falta  SnubberResistance=1e6  SnubberCapacitance=inf  Measurements=None
  Three-Phase Fault4 : powerlib/Elements/Three-Phase Fault  InitialStates=0  FaultA=on  FaultB=on  FaultC=on  GroundFault=on  SwitchTimes=[900 1000]  External=on  SwitchStatus=NaN  FaultResistance=R_falta  GroundResistance=R_falta  SnubberResistance=1e6  SnubberCapacitance=inf  Measurements=None
  Voltage Measurement : powerlib/Measurements/Voltage Measurement  PhasorSimulation=off  OutputType=Complex  PSBequivalent=0
  Voltage Measurement1 : powerlib/Measurements/Voltage Measurement  PhasorSimulation=off  OutputType=Complex  PSBequivalent=0
  Voltage Measurement2 : powerlib/Measurements/Voltage Measurement  PhasorSimulation=off  OutputType=Complex  PSBequivalent=0
  A : PMIOPort  Tag=PMCPort  Side=Right
  B : PMIOPort  Tag=PMCPort  Port=2  Side=Right
  C : PMIOPort  Tag=PMCPort  Port=3  Side=Right
  wires:
  Clock/1 -> Compare To Constant1/1
  Product2/1 -> Product3/1
  Constant1/1 -> Compare To Constant2/1
  Product/1 -> Product1/1
  Compare To Constant2/1 -> Product2/2
  Constant2/1 -> Compare To Constant4/1
  Clock2/1 -> Compare To Constant5/1
  Compare To Constant4/1 -> Product4/2
  Clock1/1 -> Compare To Constant3/1
  Compare To Constant5/1 -> Product5/2
  In1/1 -> Product/1, Product2/1, Product4/1, Product6/1
  Clock3/1 -> Compare To Constant7/1
  Constant3/1 -> Compare To Constant6/1
  Compare To Constant6/1 -> Product6/2
  Product6/1 -> Product7/1
  Compare To Constant7/1 -> Product7/2
  Compare To Constant3/1 -> Product3/2
  Constant/1 -> Compare To Constant/1
  Compare To Constant/1 -> Product/2
  Compare To Constant1/1 -> Product1/2
  Product4/1 -> Product5/1
  Product1/1 -> Product8/2
  Product8/1 -> Bistable/1
  Product3/1 -> Product9/2
  Product5/1 -> Product10/2
  Product7/1 -> Product11/2
  Compare To Constant8/1 -> Product11/1, Product10/1, Product9/1, Product8/1
  PLL (3ph)/2 -> Compare To Constant8/1
  Voltage Measurement1/1 -> Mux1/2
  Voltage Measurement/1 -> Mux1/1
  Voltage Measurement2/1 -> Mux1/3
  Mux1/1 -> PLL (3ph)/1
  Gain/1 -> Scope1/1, Three-Phase Fault1/1
  Gain1/1 -> Scope2/1, Three-Phase Fault2/1
  Gain2/1 -> Three-Phase Fault3/1, Scope3/1
  Gain3/1 -> Scope4/1, Three-Phase Fault4/1
  Bistable/1 -> Gain/1
  Product9/1 -> Bistable1/1
  Bistable1/1 -> Gain1/1
  Bistable3/1 -> Gain2/1
  Product10/1 -> Bistable3/1
  Product11/1 -> Bistable2/1
  Bistable2/1 -> Gain3/1
  connections:
  Voltage Measurement1/LConn1 -- B/RConn1 -- Three-Phase Fault1/LConn2 -- Three-Phase Fault2/LConn2 -- Three-Phase Fault3/LConn2 -- Three-Phase Fault4/LConn2
  Voltage Measurement2/LConn1 -- C/RConn1 -- Three-Phase Fault4/LConn3 -- Three-Phase Fault3/LConn3 -- Three-Phase Fault2/LConn3 -- Three-Phase Fault1/LConn3
  A/RConn1 -- Voltage Measurement/LConn1 -- Three-Phase Fault1/LConn1 -- Three-Phase Fault2/LConn1 -- Three-Phase Fault3/LConn1 -- Three-Phase Fault4/LConn1
  Ground/LConn1 -- Voltage Measurement/LConn2
  Ground1/LConn1 -- Voltage Measurement1/LConn2
  Ground2/LConn1 -- Voltage Measurement2/LConn2
